simulink model "subheart"  (R2023a)
settings: Solver=VariableStepAuto  StartTime=0.0  StopTime=120.0  RelTol=1e-3
values from neighbouring files (symbols this model uses):
  Tmin = 0.66    [Main.m]
libraries: simulink x1, simulink_extras x1
settings Model: Creator=aula  LastModifiedBy=aula

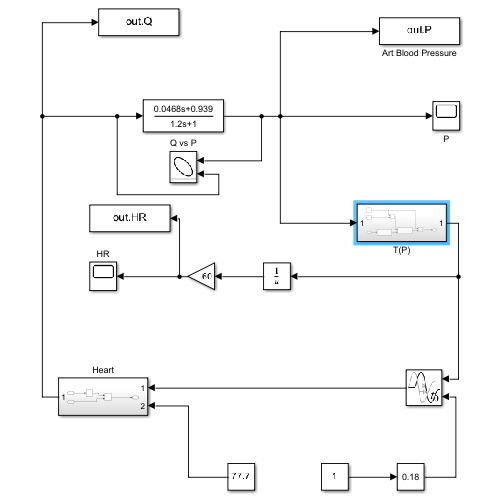
[thumbnail: Simulink's stored preview of the top-level diagram]
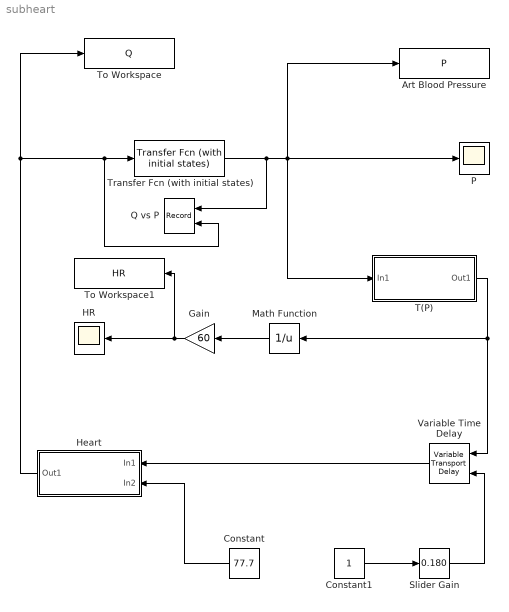
== system subheart ==
  Art Blood Pressure : ToWorkspace  VariableName=P  SaveFormat=Timeseries  SampleTime=-1
  Constant : Constant  Value=77.7
  Constant1 : Constant
  Gain : Gain  Gain=60
  HR : Scope
  Heart : Subsystem
  Math Function : Math  Operator=reciprocal
  P : Scope
  Q vs P : Record  FileSettingsInternal="{\"entries\":[{\"content\":{\"excelSettings\":{\"content\":{},\"type\":\"Streamout.ExcelSettings\"}},\"type\":\"Streamout.FileSettingStorage\",\"uuid\":\"ad8ae7e8-eaf1-4af7-a93c-93c2df4f160a\"}],\"packageUris\":[\"http://schema.mathworks.com/mf0/streamout_blocks/R2020a\"],\"version\":\"1.0\"}"  Layout=[1 1]  SignalsInternal="{\"entries\":[{\"content\":{\"signals\":[{\"content\":{\"blockPath\":[\"subheart/Q vs P\"],\"dimensions\":[1],\"domain\":\"subheart/Q vs P\",\"lineColor\":\"#ff13a6\",\"port\":1,\"sid\":[\"\"],\"signalID\":688,\"signalName\":\"Transfer Fcn\\n(with initial states)\"},\"type\":\"RecordBlkView.Signal\",\"uuid\":\"dba740f2-fb37-478b-a354-0eafcde74277\"},{\"content\":{\"blockPath\":[\"subheart/Q vs P\"],\"dimensions\":[1],\"domain\":\"subheart/Q vs P\",\"lineColor\":\"#fe330a\",\"port\":2,\"sid\":[\"\"],\"signalID\":692,\"signalName\":\"Heart\"},\"type\":\"RecordBlkView.Signal\",\"uuid\":\"549776f4-bbef-42d0-9939-c19b8d25cb99\"}]},\"type\":\"RecordBlkView.InputSignals\",\"uuid\":\"393af211-b3eb-4429-8ebe-85f037090260\"}],\"packageUris\":[\"http://schema.mathworks.com/mf0/streamout_blocks/R2020a\"],\"version\":\"1.0\"}"  VisualizationBindings="{\"xyplotplugin\":{\"info\":[{\"series\":[],\"subplotID\":1}]}}"  CompatibilityTag=XY  st=-1
  Slider Gain : simulink/Math Operations/Slider Gain  gain=0.180  low=0  high=3
  T(P) : Subsystem
  To Workspace : ToWorkspace  VariableName=Q  SaveFormat=Timeseries  SampleTime=-1
  To Workspace1 : ToWorkspace  VariableName=HR  SaveFormat=Timeseries  SampleTime=-1
  Transfer Fcn (with initial states) : simulink_extras/Additional Linear/Transfer Fcn (with initial states)  N=[0.0468 0.939]  D="[1.2  1]"  X0=100
  Variable Time Delay : VariableTransportDelay  MaximumDelay=3  InitialOutput=1
  wires:
  Transfer Fcn (with initial states)/1 -> Q vs P/1, P/1, Art Blood Pressure/1, T(P)/1(In1)
  Heart/1(Out1) -> To Workspace/1, Transfer Fcn (with initial states)/1, Q vs P/2
  Constant/1 -> Heart/2(In2)
  T(P)/1(Out1) -> Variable Time Delay/1, Math Function/1
  Math Function/1 -> Gain/1
  Variable Time Delay/1 -> Heart/1(In1)
  Constant1/1 -> Slider Gain/1
  Slider Gain/1 -> Variable Time Delay/2
  Gain/1 -> To Workspace1/1, HR/1

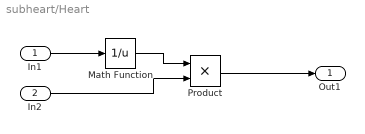
== system subheart/Heart ==
  In1 : Inport
  In2 : Inport  Port=2
  Math Function : Math  Operator=reciprocal
  Product : Product
  Out1 : Outport
  wires:
  Product/1 -> Out1/1
  In2/1 -> Product/2
  In1/1 -> Math Function/1
  Math Function/1 -> Product/1

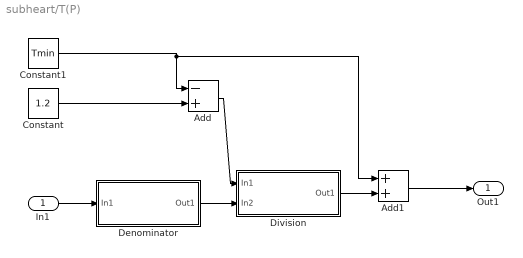
== system subheart/T(P) ==
  In1 : Inport
  Add : Sum  Inputs=-+
  Add1 : Sum
  Constant : Constant  Value=1.2
  Constant1 : Constant  Value=Tmin
  Denominator : Subsystem
  Division : Subsystem
  Out1 : Outport
  wires:
  In1/1 -> Denominator/1(In1)
  Denominator/1(Out1) -> Division/2(In2)
  Add/1 -> Division/1(In1)
  Constant/1 -> Add/2
  Constant1/1 -> Add1/1, Add/1
  Division/1(Out1) -> Add1/2
  Add1/1 -> Out1/1

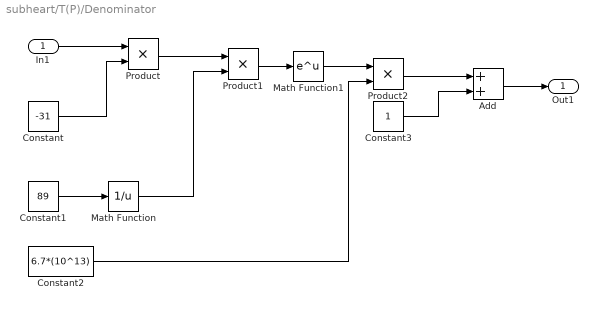
== system subheart/T(P)/Denominator ==
  In1 : Inport
  Add : Sum
  Constant : Constant  Value=-31
  Constant1 : Constant  Value=89
  Constant2 : Constant  Value=6.7*(10^13)
  Constant3 : Constant
  Math Function : Math  Operator=reciprocal
  Math Function1 : Math
  Product : Product
  Product1 : Product
  Product2 : Product
  Out1 : Outport
  wires:
  In1/1 -> Product/1
  Constant/1 -> Product/2
  Product/1 -> Product1/1
  Constant1/1 -> Math Function/1
  Math Function/1 -> Product1/2
  Product1/1 -> Math Function1/1
  Math Function1/1 -> Product2/1
  Constant2/1 -> Product2/2
  Product2/1 -> Add/1
  Constant3/1 -> Add/2
  Add/1 -> Out1/1

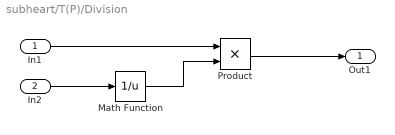
== system subheart/T(P)/Division ==
  In1 : Inport
  In2 : Inport  Port=2
  Math Function : Math  Operator=reciprocal
  Product : Product
  Out1 : Outport
  wires:
  In1/1 -> Product/1
  In2/1 -> Math Function/1
  Math Function/1 -> Product/2
  Product/1 -> Out1/1
